simulink model "test_switch_logic"  (R2022a)
settings: Solver=FixedStepAuto  StartTime=0.0  StopTime=10.0  MaxStep=1e-3  MinStep=1e-4  RelTol=1e-4
settings Model: Creator=lordx  LastModifiedBy=lordx
settings SolverCC: InitialStep=1e-4  ZeroCrossControl=EnableAll
settings OptimizationCC: OptimizeBlockIOStorage=off  EnableMemcpy=off  InitFltsAndDblsToZero=on  EfficientMapNaN2IntZero=off  BufferReusableBoundary=off
settings HardwareCC: ProdBitPerPointer=32  ProdBitPerSizeT=32  ProdBitPerPtrDiffT=32  ProdLargestAtomicFloat=None  ProdWordSize=32  ProdHWDeviceType=Altera->SoC (ARM Cortex A)  TargetBitPerPointer=64  TargetBitPerSizeT=64  TargetBitPerPtrDiffT=64  TargetLongLongMode=on  TargetIntDivRoundTo=Zero  TargetEndianess=LittleEndian  TargetWordSize=64  TargetHWDeviceType=MATLAB Host  ProdEqTarget=off
settings ModelReferenceCC: UpdateModelReferenceTargets=Force  EnableRefExpFcnMdlSchedulingChecks=off  ParallelModelReferenceMATLABWorkerInit=Load Top Model  ModelReferenceNumInstancesAllowed=Single  ModelReferenceMinAlgLoopOccurrences=on  UseModelRefSolver=on
settings RTWCC: Description=FMU based on RTW S-Function (Functional Mock-up Unit)  SystemTargetFile=rtwsfcnfmi.tlc  GenerateMakefile=off  TemplateMakefile=none  GenerateReport=on  RTWUseSimCustomCode=on  RTWCompilerOptimization=on  CheckMdlBeforeBuild=Error
settings CodeAppCC: ForceParamTrailComments=on  StateflowObjectComments=on  MATLABSourceComments=on
settings STFCustomTargetCC: TargetLangStandard=C99 (ISO)  ModelReferenceCompliant=off  CompOptLevelCompliant=on  MATLABClassNameForMDSCustomization=Simulink.SoftwareTarget.TargetSpecificTriggerConfigurationBase  SystemTargetFile=rtwsfcnfmi.tlc

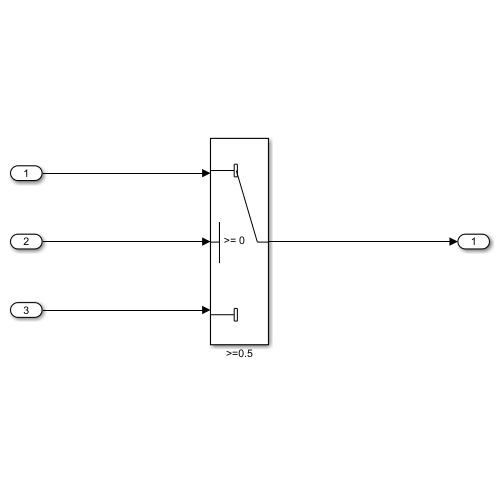
[thumbnail: Simulink's stored preview of the top-level diagram]
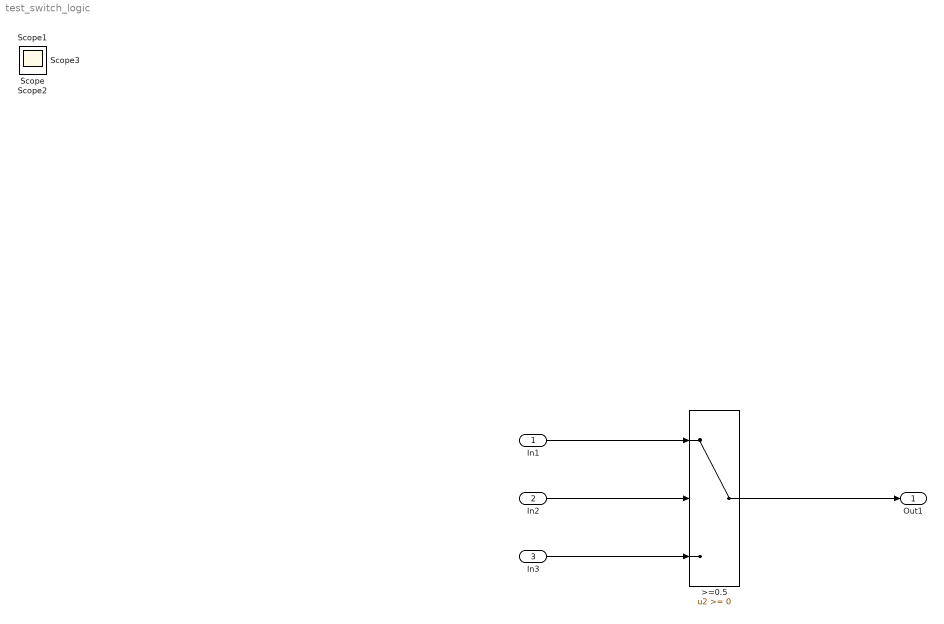
== system test_switch_logic ==
  In1 : Inport
  In2 : Inport  Port=2
  In3 : Inport  Port=3
  >=0.5 : Switch  SaturateOnIntegerOverflow=off  InputSameDT=off
  Out1 : Outport
  Scope{,1..3} (4 alike) : Scope
  wires:
  >=0.5/1 -> Out1/1
  In3/1 -> >=0.5/3
  In2/1 -> >=0.5/2
  In1/1 -> >=0.5/1
